simulink model "Edu_Read"  (R2015a)
settings: Solver=ode4  StartTime=0.0  StopTime=inf  FixedStep=0.002  RelTol=1e-3
undefined symbols (not defined in the file): Serial_Port, Standard_Devices
libraries: simulink_extras x2, vrlib x1, sldrtlib x1
settings Model: SimulationMode=external  CovSFcnEnable=off  ExtModeTrigDuration=50000  Creator=Vanya  LastModifiedBy=Ark
settings DataIOCC: SignalLoggingSaveFormat=ModelDataLogs
settings OptimizationCC: ExpressionDepthLimit=2147483647
settings DebuggingCC: UnderspecifiedInitializationDetection=Classic  MergeDetectMultiDrivingBlocksExec=none  SolverPrmCheckMsg=warning  FcnCallInpInsideContextMsg=UseLocalSettings  StateNameClashWarn=warning
settings HardwareCC: ProdBitPerLong=64  ProdBitPerPointer=64  ProdIntDivRoundTo=Zero  ProdEndianess=LittleEndian  ProdWordSize=64  ProdHWDeviceType=Intel->x86-64  TargetBitPerLong=64  TargetBitPerPointer=64  TargetIntDivRoundTo=Zero  TargetEndianess=LittleEndian  TargetWordSize=64  TargetHWDeviceType=Intel->x86-64
settings RTWCC: SystemTargetFile=rtwin.tlc  TemplateMakefile=rtwin.tmf  Description=Real-Time Windows Target  RTWCompilerOptimization=on
settings CodeAppCC: MaxIdLength=95
settings RTWinTargetCC: TargetPreCompLibLocation=C:\Program Files\MATLAB\R2015a\toolbox\sldrt\lib\win64

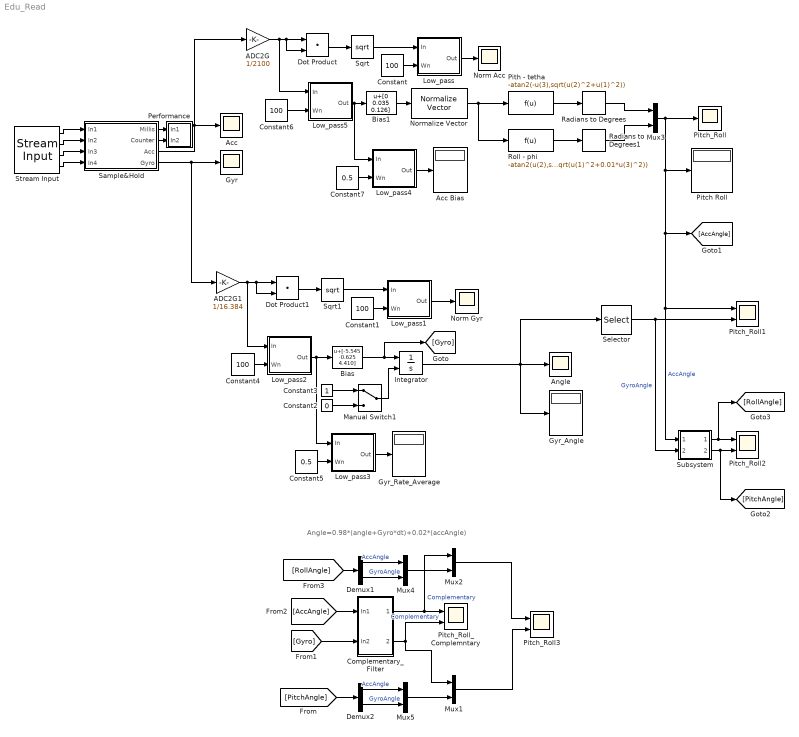
== system Edu_Read ==
  note: Angle=0.98*(angle+Gyro*dt)+0.02*(accAngle)
  ADC2G : Gain  Gain=1/2100
  ADC2G1 : Gain  Gain=1/16.384
  Acc : Scope
      settings: TimeRange=10  YMin=-8300  YMax=8300  ScrollMode=on
  Acc Bias : Display
  Angle : Scope
      settings: TimeRange=10  YMin=-720  YMax=720  SaveName=ScopeData8  ScrollMode=on
  Bias : Bias  Bias=[-5.545 -0.625 4.410]
  Bias1 : Bias  Bias=[0 0.035 0.126]
  Complementary_Filter : Subsystem
  Constant{,1,4,6} (4 alike) : Constant  Value=100
  Constant2 : Constant  Value=0
  Constant3 : Constant
  Constant5 : Constant  Value=0.5
  Constant7 : Constant  Value=0.5
  Demux1 : Demux  Outputs=2
  Demux2 : Demux  Outputs=2
  Dot Product : DotProduct  InputSameDT=on  OutDataTypeStr=Inherit: Inherit via internal rule
  Dot Product1 : DotProduct  InputSameDT=on  OutDataTypeStr=Inherit: Inherit via internal rule
  Gyr : Scope
      settings: TimeRange=10  YMin=-22500  YMax=35000  ScrollMode=on
  Gyr_Angle : Display
  Gyr_Rate_Average : Display
  Integrator : Integrator  ExternalReset=rising
  Low_pass : Subsystem
  Low_pass1 : Subsystem
  Low_pass2 : Subsystem
  Low_pass3 : Subsystem
  Low_pass4 : Subsystem
  Low_pass5 : Subsystem
  Manual Switch1 : ManualSwitch
  Mux{1..5} (5 alike) : Mux  Inputs=2
  Norm Acc : Scope
      settings: TimeRange=10  YMin=0  YMax=10  SaveName=ScopeData6  ScrollMode=on
  Norm Gyr : Scope
      settings: TimeRange=10  YMin=0  YMax=3500  SaveName=ScopeData7  ScrollMode=on
  Normalize Vector : vrlib/Utilities/Normalize Vector  maxzero=0
  Performance : Subsystem
  Pitch Roll : Display
  Pitch_Roll : Scope
      settings: YMin=-90  YMax=90  SaveName=ScopeData9  MaxDataPoints=50000
  Pitch_Roll1 : Scope  NumInputPorts=2
      settings: YMin=-180~-180  YMax=180~180  SaveName=ScopeData10  MaxDataPoints=50000  ScrollMode=on
  Pitch_Roll2 : Scope  NumInputPorts=2
      settings: YMin=-180~-180  YMax=180~180  SaveName=ScopeData11  MaxDataPoints=50000  ScrollMode=on
  Pitch_Roll3 : Scope  NumInputPorts=2
      settings: ShowLegends=on  YMin=-90~-90  YMax=90~90  SaveName=ScopeData13  MaxDataPoints=50000  ScrollMode=on
  Pitch_Roll_Complemntary : Scope  NumInputPorts=2
      settings: YMin=-180~-180  YMax=180~180  SaveName=ScopeData12  MaxDataPoints=50000  ScrollMode=on
  Pith - tetha : Fcn  Expr=-atan2(-u(3),sqrt(u(2)^2+u(1)^2))
  Radians to Degrees : simulink_extras/Transformations/Radians to Degrees
  Radians to Degrees1 : simulink_extras/Transformations/Radians to Degrees
  Roll - phi : Fcn  Expr=-atan2(u(2),sqrt(u(1)^2+0.01*u(3)^2))
  Sample&Hold : Subsystem
  Selector : Selector  InputPortWidth=3  Indices=[2 3]
  Sqrt : Sqrt  SaturateOnIntegerOverflow=on
  Sqrt1 : Sqrt  SaturateOnIntegerOverflow=on
  Stream Input : sldrtlib/Stream Input  SampleTime=0.002  MaxMissedTicks=100  ShowMissedTicks=off  YieldWhenWaiting=off  DrvName=Standard_Devices/Serial_Port  DrvAddress=17  DrvOptions=[115200 8 0 0 0 0 0 0]  DataTypes={'uint32','uint16','3*int16','3*int16'}  FormatString='MSG: %d,%d,%d,%d,%d,%d,%d,%d'  Terminator={'\r', '\n'}  ShowReady=off  ShowError=off
      settings: AttributesFormatString=Standard Devices\nSerial Port [11h]
  Subsystem : Subsystem
  wires:
  Dot Product/1 -> Sqrt/1
  Sqrt/1 -> Low_pass/1(In)
  ADC2G/1 -> Low_pass5/1(In), Dot Product/2, Dot Product/1
  Constant/1 -> Low_pass/2(Wn)
  Dot Product1/1 -> Sqrt1/1
  Sqrt1/1 -> Low_pass1/1(In)
  Constant1/1 -> Low_pass1/2(Wn)
  Low_pass1/1(Out) -> Norm Gyr/1
  Integrator/1 -> Selector/1, Gyr_Angle/1, Angle/1
  Low_pass/1(Out) -> Norm Acc/1
  ADC2G1/1 -> Low_pass2/1(In), Dot Product1/2, Dot Product1/1
  Constant4/1 -> Low_pass2/2(Wn)
  Sample&Hold/3(Acc) -> ADC2G/1, Acc/1
  Sample&Hold/4(Gyro) -> ADC2G1/1, Gyr/1
  Stream Input/1 -> Sample&Hold/1(In1)
  Stream Input/2 -> Sample&Hold/2(In2)
  Stream Input/3 -> Sample&Hold/3(In3)
  Stream Input/4 -> Sample&Hold/4(In4)
  Low_pass2/1(Out) -> Low_pass3/1(In), Bias/1
  Constant3/1 -> Manual Switch1/1
  Constant2/1 -> Manual Switch1/2
  Manual Switch1/1 -> Integrator/2
  Bias/1 -> [Gyro], Integrator/1
  Constant5/1 -> Low_pass3/2(Wn)
  Low_pass3/1(Out) -> Gyr_Rate_Average/1
  Pith - tetha/1 -> Radians to Degrees/1
  Normalize Vector/1 -> Roll - phi/1, Pith - tetha/1
  Roll - phi/1 -> Radians to Degrees1/1
  Mux3/1 -> [AccAngle], Subsystem/1(In1), Pitch_Roll1/1, Pitch Roll/1, Pitch_Roll/1  "AccAngle"
  Radians to Degrees1/1 -> Mux3/2
  Radians to Degrees/1 -> Mux3/1
  Sample&Hold/1(Millis) -> Performance/1(In1)
  Sample&Hold/2(Counter) -> Performance/2(In2)
  Constant6/1 -> Low_pass5/2(Wn)
  Low_pass5/1(Out) -> Low_pass4/1(In), Bias1/1
  Bias1/1 -> Normalize Vector/1
  Constant7/1 -> Low_pass4/2(Wn)
  Low_pass4/1(Out) -> Acc Bias/1
  Selector/1 -> Subsystem/2(In2), Pitch_Roll1/2  "GyroAngle"
  Subsystem/1(Out1) -> [RollAngle], Pitch_Roll2/1
  Subsystem/2(Out2) -> [PitchAngle], Pitch_Roll2/2
  Complementary_Filter/1(Out1) -> Mux2/1, Pitch_Roll_Complemntary/1  "Complementary"
  Complementary_Filter/2(Out2) -> Mux1/1, Pitch_Roll_Complemntary/2  "Complementary"
  [AccAngle] -> Complementary_Filter/1(In1)
  [Gyro] -> Complementary_Filter/2(In2)
  Mux1/1 -> Pitch_Roll3/2
  Mux2/1 -> Pitch_Roll3/1
  Demux1/1 -> Mux4/1  "AccAngle"
  Demux1/2 -> Mux4/2  "GyroAngle"
  Mux4/1 -> Mux2/2
  [RollAngle] -> Demux1/1
  Demux2/1 -> Mux5/1  "AccAngle"
  Demux2/2 -> Mux5/2  "GyroAngle"
  Mux5/1 -> Mux1/2
  [PitchAngle] -> Demux2/1

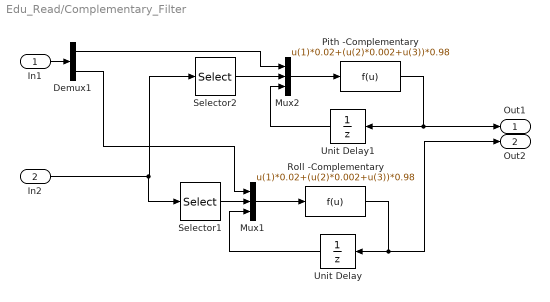
== system Edu_Read/Complementary_Filter ==
  In1 : Inport
  In2 : Inport  Port=2
  Demux1 : Demux  Outputs=2
  Mux1 : Mux  Inputs=[1 1 1]
  Mux2 : Mux  Inputs=[1 1 1]
  Pith -Complementary : Fcn  Expr=u(1)*0.02+(u(2)*0.002+u(3))*0.98
  Roll -Complementary : Fcn  Expr=u(1)*0.02+(u(2)*0.002+u(3))*0.98
  Selector1 : Selector  InputPortWidth=3  Indices=[3]
  Selector2 : Selector  InputPortWidth=3  Indices=[2]
  Unit Delay : UnitDelay  SampleTime=-1
  Unit Delay1 : UnitDelay  SampleTime=-1
  Out1 : Outport
  Out2 : Outport  Port=2
  wires:
  Selector2/1 -> Mux2/2
  Unit Delay1/1 -> Mux2/3
  Pith -Complementary/1 -> Out1/1, Unit Delay1/1
  In1/1 -> Demux1/1
  Unit Delay/1 -> Mux1/3
  Mux2/1 -> Pith -Complementary/1
  Roll -Complementary/1 -> Out2/1, Unit Delay/1
  Mux1/1 -> Roll -Complementary/1
  Selector1/1 -> Mux1/2
  In2/1 -> Selector1/1, Selector2/1
  Demux1/2 -> Mux1/1
  Demux1/1 -> Mux2/1

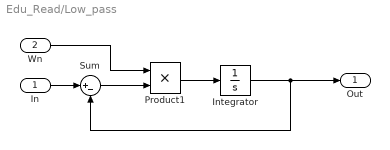
== system Edu_Read/Low_pass ==
  In : Inport
  Wn : Inport  Port=2
  Integrator : Integrator
  Product1 : Product  RndMeth=Zero
  Sum : Sum  Inputs=|+-
  Out : Outport
  wires:
  In/1 -> Sum/1
  Integrator/1 -> Out/1, Sum/2
  Sum/1 -> Product1/2
  Product1/1 -> Integrator/1
  Wn/1 -> Product1/1

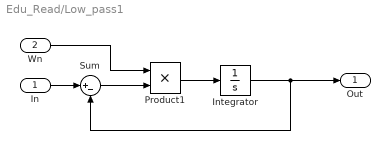
== system Edu_Read/Low_pass1 ==
  In : Inport
  Wn : Inport  Port=2
  Integrator : Integrator
  Product1 : Product  RndMeth=Zero
  Sum : Sum  Inputs=|+-
  Out : Outport
  wires:
  In/1 -> Sum/1
  Integrator/1 -> Out/1, Sum/2
  Sum/1 -> Product1/2
  Product1/1 -> Integrator/1
  Wn/1 -> Product1/1

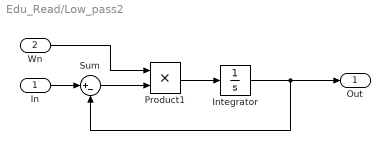
== system Edu_Read/Low_pass2 ==
  In : Inport
  Wn : Inport  Port=2
  Integrator : Integrator
  Product1 : Product  RndMeth=Zero
  Sum : Sum  Inputs=|+-
  Out : Outport
  wires:
  In/1 -> Sum/1
  Integrator/1 -> Out/1, Sum/2
  Sum/1 -> Product1/2
  Product1/1 -> Integrator/1
  Wn/1 -> Product1/1

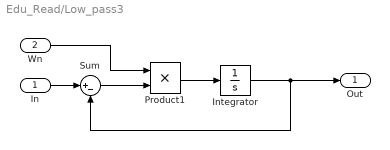
== system Edu_Read/Low_pass3 ==
  In : Inport
  Wn : Inport  Port=2
  Integrator : Integrator
  Product1 : Product  RndMeth=Zero
  Sum : Sum  Inputs=|+-
  Out : Outport
  wires:
  In/1 -> Sum/1
  Integrator/1 -> Out/1, Sum/2
  Sum/1 -> Product1/2
  Product1/1 -> Integrator/1
  Wn/1 -> Product1/1

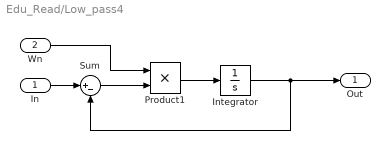
== system Edu_Read/Low_pass4 ==
  In : Inport
  Wn : Inport  Port=2
  Integrator : Integrator
  Product1 : Product  RndMeth=Zero
  Sum : Sum  Inputs=|+-
  Out : Outport
  wires:
  In/1 -> Sum/1
  Integrator/1 -> Out/1, Sum/2
  Sum/1 -> Product1/2
  Product1/1 -> Integrator/1
  Wn/1 -> Product1/1

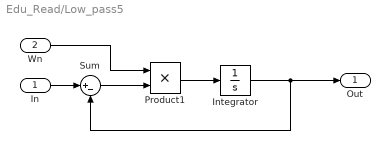
== system Edu_Read/Low_pass5 ==
  In : Inport
  Wn : Inport  Port=2
  Integrator : Integrator
  Product1 : Product  RndMeth=Zero
  Sum : Sum  Inputs=|+-
  Out : Outport
  wires:
  In/1 -> Sum/1
  Integrator/1 -> Out/1, Sum/2
  Sum/1 -> Product1/2
  Product1/1 -> Integrator/1
  Wn/1 -> Product1/1

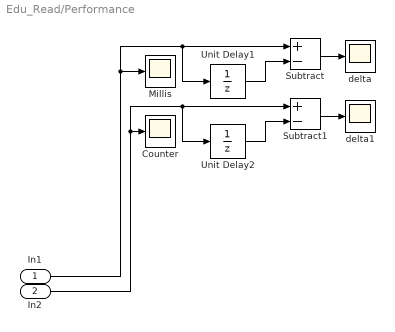
== system Edu_Read/Performance ==
  In1 : Inport
  In2 : Inport  Port=2
  Counter : Scope
      settings: TimeRange=10  YMin=1150  YMax=1800  SaveName=ScopeData3  ScrollMode=on
  Millis : Scope
      settings: TimeRange=10  YMin=3183240  YMax=3583330  SaveName=ScopeData2  ScrollMode=on
  Subtract : Sum  Inputs=+-
  Subtract1 : Sum  Inputs=+-
  Unit Delay1 : UnitDelay  SampleTime=-1
  Unit Delay2 : UnitDelay  SampleTime=-1
  delta : Scope
      settings: TimeRange=10  YMin=0  YMax=25  SaveName=ScopeData4
  delta1 : Scope
      settings: TimeRange=10  YMin=0  YMax=2  SaveName=ScopeData5  ScrollMode=on
  wires:
  Unit Delay1/1 -> Subtract/2
  Subtract/1 -> delta/1
  Unit Delay2/1 -> Subtract1/2
  Subtract1/1 -> delta1/1
  In2/1 -> Unit Delay2/1, Subtract1/1, Counter/1
  In1/1 -> Unit Delay1/1, Subtract/1, Millis/1

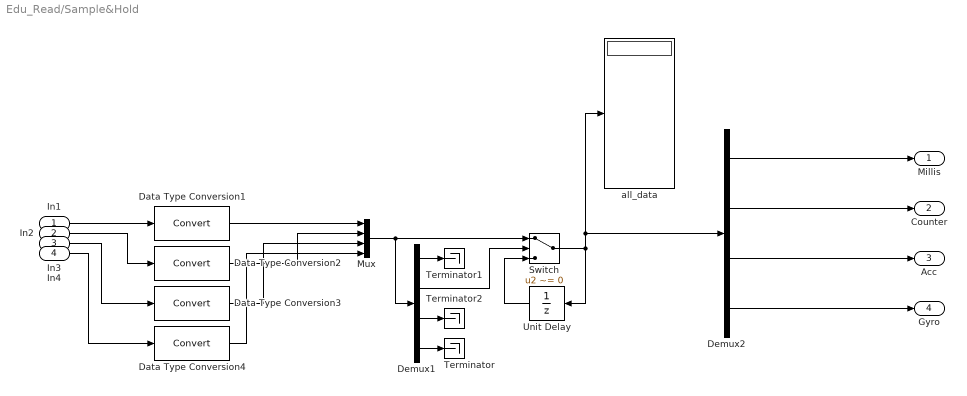
== system Edu_Read/Sample&Hold ==
  In1 : Inport
  In2 : Inport  Port=2
  In3 : Inport  Port=3
  In4 : Inport  Port=4
  Data Type Conversion{1..4} (4 alike) : DataTypeConversion
  Demux1 : Demux  Outputs=[1,1,3,3]
  Demux2 : Demux  Outputs=[1,1,3,3]
  Mux : Mux  Inputs=[1,1,3,3]
  Switch : Switch  Criteria=u2 ~= 0
  Terminator : Terminator
  Terminator1 : Terminator
  Terminator2 : Terminator
  Unit Delay : UnitDelay  SampleTime=-1
  all_data : Display
  Millis : Outport
  Counter : Outport  Port=2
  Acc : Outport  Port=3
  Gyro : Outport  Port=4
  wires:
  Demux1/4 -> Terminator/1
  Demux1/1 -> Terminator1/1
  Mux/1 -> Demux1/1, Switch/1
  Unit Delay/1 -> Switch/3
  Switch/1 -> Demux2/1, all_data/1, Unit Delay/1
  Demux1/2 -> Switch/2
  Demux2/3 -> Acc/1
  In1/1 -> Data Type Conversion1/1
  Data Type Conversion1/1 -> Mux/1
  In2/1 -> Data Type Conversion2/1
  In3/1 -> Data Type Conversion3/1
  In4/1 -> Data Type Conversion4/1
  Data Type Conversion2/1 -> Mux/2
  Data Type Conversion3/1 -> Mux/3
  Data Type Conversion4/1 -> Mux/4
  Demux2/1 -> Millis/1
  Demux2/2 -> Counter/1
  Demux2/4 -> Gyro/1
  Demux1/3 -> Terminator2/1

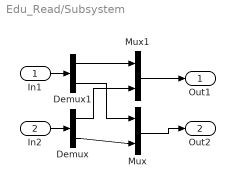
== system Edu_Read/Subsystem ==
  In1 : Inport
  In2 : Inport  Port=2
  Demux : Demux  Outputs=2
  Demux1 : Demux  Outputs=2
  Mux : Mux  Inputs=2
  Mux1 : Mux  Inputs=2
  Out1 : Outport
  Out2 : Outport  Port=2
  wires:
  In1/1 -> Demux1/1
  Demux1/2 -> Mux/1
  Mux1/1 -> Out1/1
  Demux1/1 -> Mux1/1
  In2/1 -> Demux/1
  Demux/2 -> Mux/2
  Demux/1 -> Mux1/2
  Mux/1 -> Out2/1
